simulink model "transferfunction9A_harness"  (R2022b)
settings: Solver=VariableStepAuto  StartTime=time_in(1)  StopTime=time_in(end)  FixedStep=t(2)-t(1)  MaxStep=Auto  MinStep=Auto  RelTol=1e-3
PreLoadFcn:
  | load('transferfunction9A_BaseWorkspace.mat')
settings Model: Creator=u0062516  LastModifiedBy=Kobe Michiels
settings SolverCC: InitialStep=Auto
settings DataIOCC: ExternalInput=[time_in, input]  LoadExternalInput=on  SaveFormat=Array  SignalLogging=off  DSMLogging=off  TimeSaveName=time_out  OutputSaveName=response
settings HardwareCC: TargetBitPerPointer=64  TargetBitPerSizeT=64  TargetBitPerPtrDiffT=64  TargetLongLongMode=on  TargetIntDivRoundTo=Zero  TargetEndianess=LittleEndian  TargetWordSize=64  TargetHWDeviceType=MATLAB Host  ProdEqTarget=off
settings RTWCC: Description=Rapid Simulation Target  SystemTargetFile=rsim.tlc  TemplateMakefile=rsim_default_tmf
settings CodeAppCC: GenerateComments=off
settings RSimTargetCC: TargetLangStandard=C99 (ISO)  OptimizeReductions=off

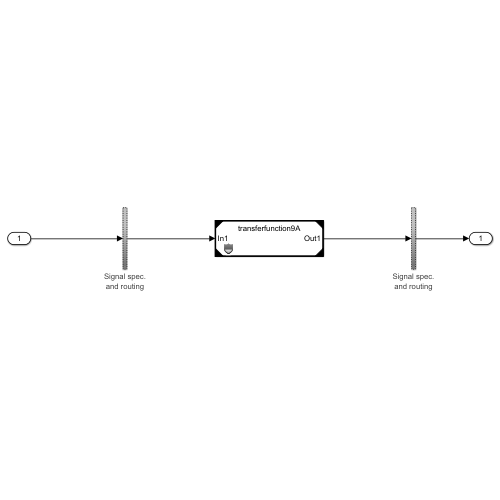
[thumbnail: Simulink's stored preview of the top-level diagram]
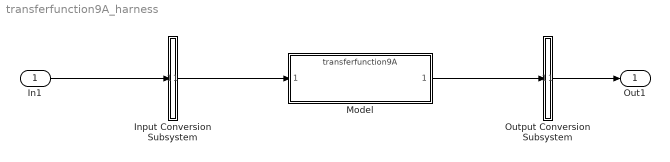
== system transferfunction9A_harness ==
  In1 : Inport  OutDataTypeStr=double  PortDimensions=[1]  SampleTime=0
  Input Conversion Subsystem : Subsystem  Tag=__SLT_ICS__  Description=|
      | Signal spec.
      | and routing
      settings: AttributesFormatString=%<Description>
  Model : ModelReference  ModelNameDialog=transferfunction9A.slxp  ModelReferenceVersion=1.38  CopyOfModelProtected=on
  Output Conversion Subsystem : Subsystem  Tag=__SLT_OCS__  Description=|
      | Signal spec.
      | and routing
      settings: AttributesFormatString=%<Description>
  Out1 : Outport
  wires:
  In1/1 -> Input Conversion Subsystem/1(Inport_1)
  Output Conversion Subsystem/1(Outport_1) -> Out1/1
  Input Conversion Subsystem/1(Outport_1) -> Model/1
  Model/1 -> Output Conversion Subsystem/1(Inport_1)

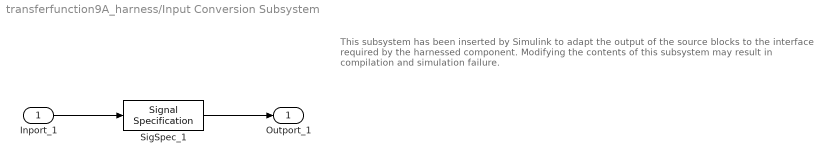
== system transferfunction9A_harness/Input Conversion Subsystem ==
  note: This subsystem has been inserted by Simulink to adapt the output of the source blocks to the interface required by the harnessed component.
      |  Modifying the contents of this subsystem may result in compilation and simulation failure.
  Inport_1 : Inport
  SigSpec_1 : SignalSpecification  OutDataTypeStr=double  Dimensions=[1]  SampleTime=[0, 0]
  Outport_1 : Outport
  wires:
  SigSpec_1/1 -> Outport_1/1
  Inport_1/1 -> SigSpec_1/1

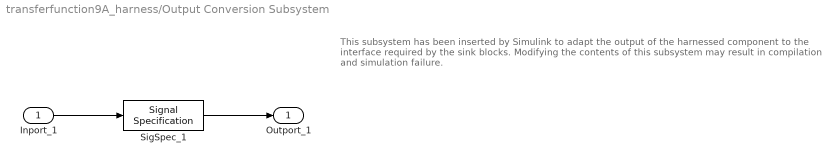
== system transferfunction9A_harness/Output Conversion Subsystem ==
  note: This subsystem has been inserted by Simulink to adapt the output of the harnessed component to the interface required by the sink blocks.
      |  Modifying the contents of this subsystem may result in compilation and simulation failure.
  Inport_1 : Inport
  SigSpec_1 : SignalSpecification  OutDataTypeStr=double  Dimensions=[1]
  Outport_1 : Outport
  wires:
  Inport_1/1 -> SigSpec_1/1
  SigSpec_1/1 -> Outport_1/1
